simulink model "proc_control"  (R2024b)
settings: Solver=FixedStepAuto  StartTime=0.0  StopTime=inf  RelTol=1e-3
InitFcn:
  | InitProcControl;
model workspace (MAT data in the model file):
  SL_ROS_VariableLengthArrays_MaxSizes : object (value not decoded)
values from neighbouring files (symbols this model uses):
  A = T200Spec16V{:,3}    [InitProcControl.m]
  dmax = simulation.drift.nominal .* rand(1,6)    [InitProcControl.m]
  dmin = -simulation.drift.nominal .* rand(1,6)    [InitProcControl.m]
  dSeedX = round(rand*10)    [InitProcControl.m]
  dts = 5    [InitProcControl.m]
  N = T200Spec16V{:,6}    [InitProcControl.m]
  PWM = T200Spec16V{:,1}    [InitProcControl.m]
  RPM = T200Spec16V{:,2}    [InitProcControl.m]
undefined symbols (not defined in the file or in its folder): angular_velocity, current_gains, data, data_SL_Info, DiscIntNeverNeededParam, elevation, heading, is_mpc_alive, is_trajectory_done, linear_acceleration, motor1, motor2, motor3, motor4, motor5, motor6, motor7, motor8, MPC, mpc_mode, mpc_status, orientation, physics, pose, position, simulation, simulink, target_reached, thrusters_status, thrusters_status_SL_Info, twist, x_vel_btm, y_vel_btm, z_vel_btm
libraries: ros2lib x85, aerolibutil x12, simulink x9, mpclib x3, embmathops x2, sharedtransform x2, robotcorelib x2, sharedTrackingLibrary x1
(part 3 of 3)

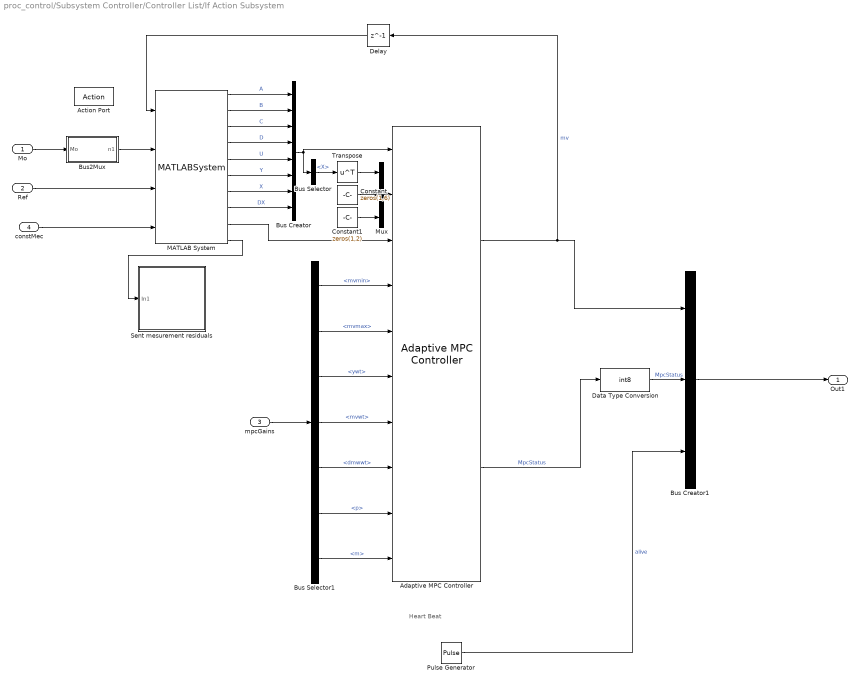
== system proc_control/Subsystem Controller/Controller List/If Action Subsystem ==
  note: Heart Beat
  Mo : Inport
  Ref : Inport  Port=2
  mpcGains : Inport  Port=3
  constMec : Inport  Port=4
  Action Port : ActionPort  InitializeStates=reset  PropagateVarSize=During execution  ActionPortLabel=case [ 10 11 19 31 ]:
  Adaptive MPC Controller : mpclib/Adaptive MPC Controller  SCDEnableBlockLinearizationSpecification=on  mpcobj=Qmpcobj  enable_value=0  updateMPCinCallerWorkspace=on  md_inport=off  mv_inport=off  uref_inport=off  return_cost=off  return_mvseq=off  return_qpstatus=on  return_xseq=off  return_state=off  return_ovseq=off  state_inport=on  isltv_plant=off  umin_inport=on  umax_inport=on  ymin_inport=off  ymax_inport=off  cc_inport=off  ywt_inport=on  uwt_inport=on  duwt_inport=on  rhoeps_inport=off  pm_inport=on  MaximumP=10  HorizonChoice=VariableHorizon  BlockDataType=double  SampleTimeInherited=off  switch_inport=off
  Bus Creator : BusCreator  Inputs=8
  Bus Creator1 : BusCreator  Inputs=3
  Bus Selector : BusSelector  OutputSignals=X
  Bus Selector1 : BusSelector  OutputSignals=mvmin,mvmax,ywt,mvwt,dmwwt,p,m
  Bus2Mux : Subsystem
  Constant : Constant  Value=zeros(1,6)
  Constant1 : Constant  Value=zeros(1,2)
  Data Type Conversion : DataTypeConversion  OutDataTypeStr=int8  SaturateOnIntegerOverflow=off  RndMeth=Floor
  Delay : Delay  DelayLength=1  InitialCondition=zeros(MPC.nu,1)  SampleTime=MPC.Ts
  MATLAB System : MATLABSystem  System=TrimPlant  MPC=MPC  useDynamicsConst=on  SimulateUsing=Code generation
      mask Type: TrimPlant
      mask Display:
      | disp('TrimPlant');
      | port_label('input',1,'u');
      | port_label('input',2,'y');
      | port_label('input',3,'ref');
      | port_label('input',4,'constMec');
      | port_label('output',1,'A');
      | port_label('output',2,'B');
      | port_label('output',3,'C');
      | port_label('output',4,'D');
      | port_label('output',5,'U');
      | port_label('output',6,'Y');
      | port_label('output',7,'X');
      | port_label('output',8,'DX');
      | port_label('output',9,'ref');
      | port_label('output',10,'Z');
  Mux : Mux  Inputs=3
  Pulse Generator : DiscretePulseGenerator  SampleTime=MPC.Ts
  Sent mesurement residuals : Subsystem
  Transpose : Math  Operator=transpose
  Out1 : Outport
  wires:
  Mo/1 -> Bus2Mux/1(Mo)
  Bus2Mux/1(n1) -> MATLAB System/2
  Ref/1 -> MATLAB System/3
  constMec/1 -> MATLAB System/4
  MATLAB System/1 -> Bus Creator/1  "A"
  MATLAB System/2 -> Bus Creator/2  "B"
  MATLAB System/3 -> Bus Creator/3  "C"
  MATLAB System/4 -> Bus Creator/4  "D"
  MATLAB System/5 -> Bus Creator/5  "U"
  MATLAB System/6 -> Bus Creator/6  "Y"
  MATLAB System/7 -> Bus Creator/7  "X"
  MATLAB System/8 -> Bus Creator/8  "DX"
  Bus Creator/1 -> Bus Selector/1, Adaptive MPC Controller/1
  Constant/1 -> Mux/2
  Constant1/1 -> Mux/3
  Mux/1 -> Adaptive MPC Controller/2
  Bus Selector/1 -> Transpose/1  "<X>"
  Transpose/1 -> Mux/1
  MATLAB System/9 -> Adaptive MPC Controller/3
  mpcGains/1 -> Bus Selector1/1
  Bus Selector1/1 -> Adaptive MPC Controller/4  "<mvmin>"
  Bus Selector1/2 -> Adaptive MPC Controller/5  "<mvmax>"
  Bus Selector1/3 -> Adaptive MPC Controller/6  "<ywt>"
  Bus Selector1/4 -> Adaptive MPC Controller/7  "<mvwt>"
  Bus Selector1/5 -> Adaptive MPC Controller/8  "<dmwwt>"
  Bus Selector1/6 -> Adaptive MPC Controller/9  "<p>"
  Bus Selector1/7 -> Adaptive MPC Controller/10  "<m>"
  MATLAB System/10 -> Sent mesurement residuals/1(In1)
  Adaptive MPC Controller/1 -> Delay/1, Bus Creator1/1  "mv"
  Adaptive MPC Controller/2 -> Data Type Conversion/1  "MpcStatus"
  Pulse Generator/1 -> Bus Creator1/3  "alive"
  Delay/1 -> MATLAB System/1
  Bus Creator1/1 -> Out1/1
  Data Type Conversion/1 -> Bus Creator1/2  "MpcStatus"

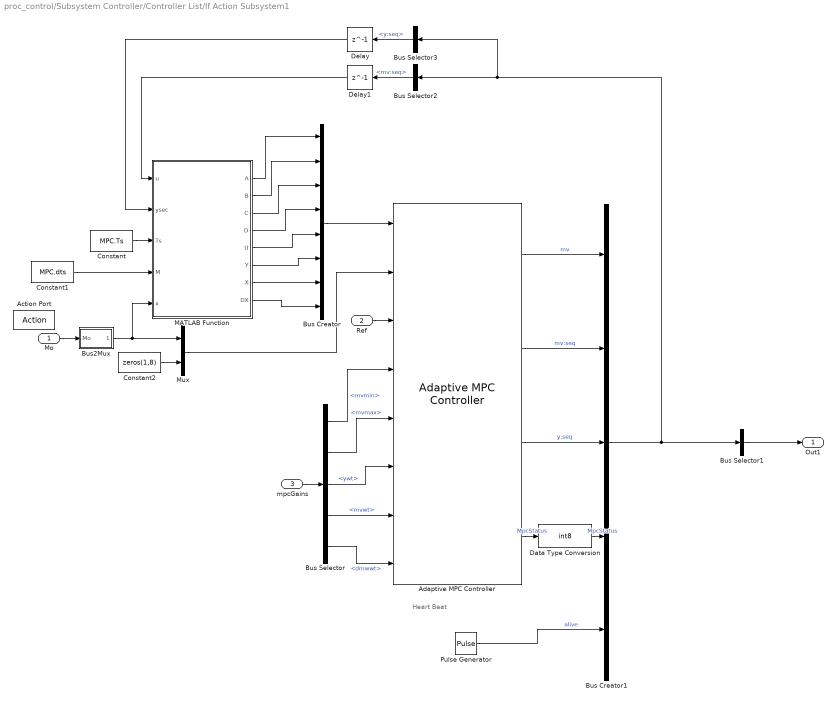
== system proc_control/Subsystem Controller/Controller List/If Action Subsystem1 ==
  note: Heart Beat
  Mo : Inport
  Ref : Inport  Port=2
  mpcGains : Inport  Port=3
  Action Port : ActionPort  InitializeStates=reset  PropagateVarSize=During execution  ActionPortLabel=case [ 30 ]:
  Adaptive MPC Controller : mpclib/Adaptive MPC Controller  SCDEnableBlockLinearizationSpecification=on  mpcobj=Qmpcobj  enable_value=0  updateMPCinCallerWorkspace=on  md_inport=off  mv_inport=off  uref_inport=off  return_cost=off  return_mvseq=on  return_qpstatus=on  return_xseq=off  return_state=off  return_ovseq=on  state_inport=on  isltv_plant=on  umin_inport=on  umax_inport=on  ymin_inport=off  ymax_inport=off  cc_inport=off  ywt_inport=on  uwt_inport=on  duwt_inport=on  rhoeps_inport=off  pm_inport=off  MaximumP=10  HorizonChoice=FixedHorizon  BlockDataType=double  SampleTimeInherited=off  switch_inport=off
  Bus Creator : BusCreator  Inputs=8
  Bus Creator1 : BusCreator  Inputs=5
  Bus Selector : BusSelector  OutputSignals=mvmin,mvmax,ywt,mvwt,dmwwt
  Bus Selector1 : BusSelector  OutputSignals=mv,MpcStatus,alive  OutputAsBus=on
  Bus Selector2 : BusSelector  OutputSignals=mv:seq
  Bus Selector3 : BusSelector  OutputSignals=y:seq
  Bus2Mux : Subsystem
  Constant : Constant  Value=MPC.Ts
  Constant1 : Constant  Value=MPC.dts
  Constant2 : Constant  Value=zeros(1,8)
  Data Type Conversion : DataTypeConversion  OutDataTypeStr=int8  SaturateOnIntegerOverflow=off  RndMeth=Floor
  Delay : Delay  DelayLength=1  InitialCondition=repmat(MPC.Xi.',11,1)  SampleTime=MPC.Ts
  Delay1 : Delay  DelayLength=1  InitialCondition=zeros(11,8)  SampleTime=MPC.Ts
  MATLAB Function : MATLAB Function  TreatAsAtomicUnit=on
  Mux : Mux  Inputs=2
  Pulse Generator : DiscretePulseGenerator  SampleTime=MPC.Ts
  Out1 : Outport
  wires:
  MATLAB Function/2(B) -> Bus Creator/2
  Mo/1 -> Bus2Mux/1(Mo)
  Constant/1 -> MATLAB Function/3(Ts)
  Constant1/1 -> MATLAB Function/4(M)
  Bus Selector/5 -> Adaptive MPC Controller/8  "<dmwwt>"
  MATLAB Function/7(X) -> Bus Creator/7
  Bus2Mux/1(Out1) -> Mux/1, MATLAB Function/5(x)
  Constant2/1 -> Mux/2
  MATLAB Function/3(C) -> Bus Creator/3
  MATLAB Function/1(A) -> Bus Creator/1
  Ref/1 -> Adaptive MPC Controller/3
  Mux/1 -> Adaptive MPC Controller/2
  MATLAB Function/4(D) -> Bus Creator/4
  MATLAB Function/5(U) -> Bus Creator/5
  MATLAB Function/6(Y) -> Bus Creator/6
  MATLAB Function/8(DX) -> Bus Creator/8
  mpcGains/1 -> Bus Selector/1
  Bus Creator/1 -> Adaptive MPC Controller/1
  Bus Selector/2 -> Adaptive MPC Controller/5  "<mvmax>"
  Bus Selector/1 -> Adaptive MPC Controller/4  "<mvmin>"
  Bus Selector/3 -> Adaptive MPC Controller/6  "<ywt>"
  Bus Selector/4 -> Adaptive MPC Controller/7  "<mvwt>"
  Adaptive MPC Controller/1 -> Bus Creator1/1  "mv"
  Adaptive MPC Controller/4 -> Data Type Conversion/1  "MpcStatus"
  Adaptive MPC Controller/3 -> Bus Creator1/3  "y:seq"
  Adaptive MPC Controller/2 -> Bus Creator1/2  "mv:seq"
  Pulse Generator/1 -> Bus Creator1/5  "alive"
  Bus Selector1/1 -> Out1/1
  Bus Creator1/1 -> Bus Selector3/1, Bus Selector2/1, Bus Selector1/1
  Bus Selector3/1 -> Delay/1  "<y:seq>"
  Bus Selector2/1 -> Delay1/1  "<mv:seq>"
  Delay1/1 -> MATLAB Function/1(u)
  Delay/1 -> MATLAB Function/2(ysec)
  Data Type Conversion/1 -> Bus Creator1/4  "MpcStatus"

== system proc_control/Subsystem Controller/Controller List/If Action Subsystem2 ==
  mo : Inport
  ref : Inport  Port=2
  mode : Inport  Port=3
  Action Port : ActionPort  ActionPortLabel=case [ 20 21 ]:
  Bus Creator : BusCreator  Inputs=3
  Constant : Constant  Value=int8(0)
  Constant1 : Constant  Value=0
  Discrete Derivative : simulink/Discrete/Discrete Derivative  gainval=1.0  ICPrevScaledInput=0.0  OutMin=[]  OutMax=[]  OutDataType=fixdt(1, 16)  OutScaling=2^-10  DoSatur=off
  MATLAB System : MATLABSystem  System=OpenLoopController  k=40  binv=binv  mass=physics.mass  volume=physics.volume  height=physics.height  I=physics.I  RG=physics.RG  RB=physics.RB  AddedMass=physics.AddedMass  CDL=physics.CDL  CDQ=physics.CDQ  AF=physics.AF  g=physics.g  rho=physics.rho  SimulateUsing=Code generation
      mask Type: OpenLoopController
      mask Display:
      | disp('OpenLoopController');
      | port_label('input',1,'ref');
      | port_label('input',2,'ref_dot');
      | port_label('input',3,'mo');
      | port_label('input',4,'mode');
      | port_label('output',1,'mv');
  Reshape : Reshape
  Selector : Selector  NumberOfDimensions=2  InputPortWidth=3  IndexOptions=Index vector (dialog),Index vector (dialog)  Indices=1,[8:13]  OutputSizes=1,1
  Out1 : Outport
  wires:
  mode/1 -> MATLAB System/4
  ref/1 -> Selector/1
  Selector/1 -> MATLAB System/1, Discrete Derivative/1
  Discrete Derivative/1 -> MATLAB System/2
  Reshape/1 -> Bus Creator/1  "mv"
  MATLAB System/1 -> Reshape/1
  mo/1 -> MATLAB System/3
  Constant/1 -> Bus Creator/2  "MpcStatus"
  Constant1/1 -> Bus Creator/3  "alive"
  Bus Creator/1 -> Out1/1

== system proc_control/Subsystem Controller/Controller List/If Action Subsystem3 ==
  Action Port : ActionPort  ActionPortLabel=default:
  Bus Creator : BusCreator  Inputs=3
  Constant : Constant  Value=zeros(1,MPC.nu)
  Constant1 : Constant  Value=int8(0)
  Constant2 : Constant  Value=0
  Out1 : Outport
  wires:
  Constant/1 -> Bus Creator/1  "mv"
  Constant1/1 -> Bus Creator/2  "MpcStatus"
  Constant2/1 -> Bus Creator/3  "alive"
  Bus Creator/1 -> Out1/1

== system proc_control/Subsystem Controller/Controller List/Quaternion Non linear MPC (Not for codegen) ==
  note: Heart beat
  Mo : Inport
  Ref : Inport  Port=2
  mpc Gains : Inport  Port=3
  Action Port : ActionPort  InitializeStates=reset  ActionPortLabel=case [ 40 ]:
  Bus Creator : BusCreator  Inputs=3
  Bus Selector : BusSelector  OutputSignals=mvmin,mvmax,ywt,mvwt,dmwwt
  Bus2Mux1 : Subsystem
  Data Type Conversion : DataTypeConversion  OutDataTypeStr=int8  SaturateOnIntegerOverflow=off  RndMeth=Floor
  Delay : Delay  DelayLength=1  InitialCondition=zeros(MPC.nu,1)
  Nonlinear MPC Controller : mpclib/Nonlinear MPC Controller  nlmpcobj=nlobj  UseObjectTs=on  TsControl=0.02  UseMEX=off  md_enabled=off  mvtarget_enabled=off  param_enabled=off  cost_enabled=off  mvseq_enabled=off  stateseq_enabled=off  ovseq_enabled=off  slack_enabled=off  status_enabled=on  ov_min=off  ov_max=off  mv_min=on  mv_max=on  mvrate_min=off  mvrate_max=off  state_min=off  state_max=off  ov_weight=on  mv_weight=on  mvrate_weight=on  ecr_weight=off  nlp_initialize=off
  Pulse Generator : DiscretePulseGenerator  Period=20  PulseWidth=10  SampleTime=MPC.Ts
  Out : Outport
  wires:
  Mo/1 -> Bus2Mux1/1(Mo)
  Bus2Mux1/1(Out1) -> Nonlinear MPC Controller/1
  Ref/1 -> Nonlinear MPC Controller/2
  mpc Gains/1 -> Bus Selector/1
  Bus Selector/1 -> Nonlinear MPC Controller/4  "<mvmin>"
  Bus Selector/2 -> Nonlinear MPC Controller/5  "<mvmax>"
  Bus Selector/3 -> Nonlinear MPC Controller/6  "<ywt>"
  Bus Selector/4 -> Nonlinear MPC Controller/7  "<mvwt>"
  Bus Selector/5 -> Nonlinear MPC Controller/8  "<dmwwt>"
  Nonlinear MPC Controller/1 -> Bus Creator/1, Delay/1  "mv"
  Delay/1 -> Nonlinear MPC Controller/3
  Nonlinear MPC Controller/2 -> Data Type Conversion/1  "MpcStatus"
  Pulse Generator/1 -> Bus Creator/3  "alive"
  Bus Creator/1 -> Out/1
  Data Type Conversion/1 -> Bus Creator/2  "MpcStatus"

== system proc_control/Subsystem Controller/If Action Subsystem/Subsystem ==
  Bus Creator : BusCreator  Inputs=8
  Constant : Constant  Value=zeros(1, 128)
  Constant1 : Constant  Value=zeros(1, 128)
  Constant2 : Constant  Value=zeros(1, 128)
  Constant3 : Constant  Value=MPC.tmax
  Constant4 : Constant  Value=MPC.tmin
  Subsystem : Subsystem
  Subsystem1 : Subsystem
  Subsystem2 : Subsystem
  Out1 : Outport
  wires:
  Constant4/1 -> Bus Creator/8  "min_thrust"
  Constant2/1 -> Bus Creator/5  "mvr"
  Constant3/1 -> Bus Creator/7  "max_thrust"
  Constant/1 -> Bus Creator/1  "ov"
  Subsystem/1(Out1) -> Bus Creator/2  "ov_SL_Info"
  Subsystem2/1(Out1) -> Bus Creator/4  "mv_SL_Info"
  Constant1/1 -> Bus Creator/3  "mv"
  Subsystem1/1(Out1) -> Bus Creator/6  "mvr_SL_Info"
  Bus Creator/1 -> Out1/1

== system proc_control/Subsystem ProcNav/DVL Measurements/DVL2Ship ==
  dvl Rotation : Inport
  Constant : Constant  Value=0
  Delay : Delay  DelayLength=1  InitialCondition=1
  Enabled Subsystem : Subsystem  TreatAsAtomicUnit=on
  Quat : Outport
  wires:
  Constant/1 -> Delay/1
  Delay/1 -> Enabled Subsystem/Enable
  dvl Rotation/1 -> Enabled Subsystem/1(dvl Rotation)
  Enabled Subsystem/1(Quat) -> Quat/1

== system proc_control/Subsystem ProcNav/SLAM Measurements/Subsystem ==
  VisData : Inport
  Blank Message : ros2lib/Blank Message  messageClass=Message  entityType=nav_msgs/Odometry  messageType=nav_msgs/Odometry  SampleTime=inf
  Bus Assignment : BusAssignment  AssignedSignals=pose.pose.position.x,pose.pose.position.y,pose.pose.position.z,pose.pose.orientation.w,pose.pose.orientation.x,pose.pose.orientation.y,pose.pose.orientation.z,twist.twist.linear.x,twist.twist.linear.y,twist.twist.linear.z,twist.twist.angular.x,twist.twist.angular.y,twist.twist.angular.z
  Demux : Demux  Outputs=13
  Header Assignment : ros2lib/Header Assignment  SetFrameID=off  InsertTimeStamp=on  SetHeaderFieldName=Use the default header field name  HeaderFieldName=header
  Publish : ros2lib/Publish  topicSource=Specify your own  topic=/proc_nav/slam/vis  messageType=nav_msgs/Odometry  QOSHistory=Keep last  QOSDepth=1  QOSReliability=Reliable  QOSDurability=Volatile  QOSDeadline=Inf  QOSLifespan=Inf  QOSLiveliness=Automatic  QOSLeaseDuration=Inf  QOSAvoidROSNamespaceConventions=off
  wires:
  Demux/8 -> Bus Assignment/9
  Demux/10 -> Bus Assignment/11
  Blank Message/1 -> Header Assignment/1
  Demux/6 -> Bus Assignment/7
  Demux/2 -> Bus Assignment/3
  Bus Assignment/1 -> Publish/1
  Demux/9 -> Bus Assignment/10
  Demux/13 -> Bus Assignment/14
  Demux/5 -> Bus Assignment/6
  Demux/7 -> Bus Assignment/8
  VisData/1 -> Demux/1
  Demux/3 -> Bus Assignment/4
  Header Assignment/1 -> Bus Assignment/1
  Demux/4 -> Bus Assignment/5
  Demux/12 -> Bus Assignment/13
  Demux/1 -> Bus Assignment/2
  Demux/11 -> Bus Assignment/12

== system proc_control/Subsystem ProcNav/SLAM Measurements/Subsystem1 ==
  TrackingData : Inport
  Blank Message : ros2lib/Blank Message  messageClass=Message  entityType=nav_msgs/Odometry  messageType=nav_msgs/Odometry  SampleTime=inf
  Bus Assignment : BusAssignment  AssignedSignals=pose.pose.position.x,pose.pose.position.y,pose.pose.position.z,pose.pose.orientation.w,pose.pose.orientation.x,pose.pose.orientation.y,pose.pose.orientation.z,twist.twist.linear.x,twist.twist.linear.y,twist.twist.linear.z,twist.twist.angular.x,twist.twist.angular.y,twist.twist.angular.z
  Demux : Demux  Outputs=13
  Header Assignment : ros2lib/Header Assignment  SetFrameID=off  InsertTimeStamp=on  SetHeaderFieldName=Use the default header field name  HeaderFieldName=header
  Publish : ros2lib/Publish  topicSource=Specify your own  topic=/proc_nav/slam/tracking  messageType=nav_msgs/Odometry  QOSHistory=Keep last  QOSDepth=1  QOSReliability=Reliable  QOSDurability=Volatile  QOSDeadline=Inf  QOSLifespan=Inf  QOSLiveliness=Automatic  QOSLeaseDuration=Inf  QOSAvoidROSNamespaceConventions=off
  wires:
  Demux/8 -> Bus Assignment/9
  Demux/10 -> Bus Assignment/11
  Blank Message/1 -> Header Assignment/1
  Demux/6 -> Bus Assignment/7
  Demux/2 -> Bus Assignment/3
  Bus Assignment/1 -> Publish/1
  Demux/9 -> Bus Assignment/10
  Demux/13 -> Bus Assignment/14
  Demux/5 -> Bus Assignment/6
  Demux/7 -> Bus Assignment/8
  TrackingData/1 -> Demux/1
  Demux/3 -> Bus Assignment/4
  Header Assignment/1 -> Bus Assignment/1
  Demux/4 -> Bus Assignment/5
  Demux/12 -> Bus Assignment/13
  Demux/1 -> Bus Assignment/2
  Demux/11 -> Bus Assignment/12

== system proc_control/Subsystem Trajectory/singleWpts Trajectory Control DEBUG only/Enabled Subsystem ==
  In1 : Inport
  Enable : EnablePort
  Bus Selector : BusSelector  OutputSignals=frame,speed  OutputAsBus=on
  Bus Selector1 : BusSelector  OutputSignals=position.x,position.y,position.z,orientation.z,orientation.y,orientation.x  OutputAsBus=on
  Bus Selector2 : BusSelector  OutputSignals=fine  OutputAsBus=on
  Data Type Conversion : DataTypeConversion  OutDataTypeStr=double  SaturateOnIntegerOverflow=off  RndMeth=Floor  LockScale=on
  Data Type Conversion1 : DataTypeConversion  OutDataTypeStr=double  SaturateOnIntegerOverflow=off  RndMeth=Floor  LockScale=on
  Data Type Conversion2 : DataTypeConversion  OutDataTypeStr=double  SaturateOnIntegerOverflow=off  RndMeth=Floor  LockScale=on
  Mux : Mux  Inputs=3
  Out1 : Outport
  wires:
  In1/1 -> Bus Selector2/1, Bus Selector1/1, Bus Selector/1
  Bus Selector1/1 -> Data Type Conversion/1
  Bus Selector2/1 -> Data Type Conversion2/1
  Bus Selector/1 -> Data Type Conversion1/1
  Mux/1 -> Out1/1
  Data Type Conversion/1 -> Mux/1
  Data Type Conversion1/1 -> Mux/2
  Data Type Conversion2/1 -> Mux/3

== system proc_control/Subsystem Trajectory/singleWpts Trajectory Control DEBUG only/Pre-traitement ==
  In1 : Inport
  Enable : EnablePort
  Constant : Constant  Value=0
  Display : Display
  Matrix Concatenate : Concatenate  Mode=Multidimensional array
  Selector : Selector  NumberOfDimensions=2  InputPortWidth=3  IndexOptions=Index vector (dialog),Index vector (dialog)  Indices=[1:3],[1:2]  OutputSizes=1,1
  Selector1 : Selector  NumberOfDimensions=2  InputPortWidth=3  IndexOptions=Index vector (dialog),Index vector (dialog)  Indices=[4:7],[1:2]  OutputSizes=1,1
  Selector2 : Selector  NumberOfDimensions=2  InputPortWidth=3  IndexOptions=Index vector (dialog),Index vector (dialog)  Indices=[8],[2]  OutputSizes=1,1
  Selector3 : Selector  NumberOfDimensions=2  InputPortWidth=3  IndexOptions=Index vector (dialog),Index vector (dialog)  Indices=[9],[2]  OutputSizes=1,1
  Selector4 : Selector  NumberOfDimensions=2  InputPortWidth=3  IndexOptions=Index vector (dialog),Index vector (dialog)  Indices=[1:7],[2]  OutputSizes=1,1
  Terminator : Terminator
  Transpose : Math  Operator=transpose
  linWpts : Outport
  RotWpts : Outport  Port=2
  time : Outport  Port=3
  target : Outport  Port=4
  wires:
  In1/1 -> Transpose/1
  Transpose/1 -> Display/1, Selector4/1, Selector3/1, Selector2/1, Selector1/1, Selector/1
  Selector/1 -> linWpts/1
  Selector1/1 -> RotWpts/1
  Constant/1 -> Matrix Concatenate/1
  Selector2/1 -> Matrix Concatenate/2
  Matrix Concatenate/1 -> time/1
  Selector3/1 -> Terminator/1
  Selector4/1 -> target/1

== system proc_control/Subsystem Trajectory/singleWpts Trajectory Control DEBUG only/Resettable Subsystem ==
  linWpts : Inport
  rotWpts : Inport  Port=2
  time : Inport  Port=3
  Reset : ResetPort  DisableCoverage=on
  Constant : Constant
  Discrete-Time Integrator : DiscreteIntegrator  IntegratorMethod=Integration: Trapezoidal  SampleTime=-1  ICPrevOutput=DiscIntNeverNeededParam  ICPrevScaledInput=DiscIntNeverNeededParam
  Rotation Trajectory : robotcorelib/Rotation Trajectory  WaypointFormat=Quaternion  WaypointSource=External  R0=[ 1, 0, 0, 0 ]'  RF=[ 0, 0, 1, 0 ]'  TimeInterval=[ 0, 1 ]  CustomTimeScaling=off  ParameterSource=Internal  TSTime=0:0.1:1  TimeScaling=[ 0:0.1:1; ones( 1, 11 ); zeros( 1, 11 ) ]  SimulateUsing=Code generation
      settings: LibrarySourceBlock=robotutilslib/Rotation Trajectory
  Selector : Selector  NumberOfDimensions=2  InputPortWidth=3  IndexOptions=Index vector (dialog),Index vector (dialog)  Indices=[1:4],1  OutputSizes=1,1
  Selector1 : Selector  NumberOfDimensions=2  InputPortWidth=3  IndexOptions=Index vector (dialog),Index vector (dialog)  Indices=[1:4],1  OutputSizes=1,1
  Subsystem : Subsystem
  Terminator : Terminator
  n1 : Outport
  epsilon : Outport  Port=2
  v1 : Outport  Port=3
  v2 : Outport  Port=4
  wires:
  Rotation Trajectory/3 -> Terminator/1
  time/1 -> Subsystem/3(time), Rotation Trajectory/4
  Constant/1 -> Discrete-Time Integrator/1
  linWpts/1 -> Subsystem/2(linWpts)
  Rotation Trajectory/1 -> epsilon/1
  Selector1/1 -> Rotation Trajectory/3
  Subsystem/1(n1) -> n1/1
  rotWpts/1 -> Selector1/1, Selector/1
  Discrete-Time Integrator/1 -> Rotation Trajectory/1, Subsystem/1(In1)
  Rotation Trajectory/2 -> v2/1
  Selector/1 -> Rotation Trajectory/2
  Subsystem/2(v1) -> v1/1

== system proc_control/Subsystem Trajectory/singleWpts Trajectory Control DEBUG only/Subsystem ==
  Bus Creator : BusCreator  Inputs=3
  Bus Creator1 : BusCreator  Inputs=3
  Bus Creator2 : BusCreator  Inputs=6
  Constant{1..6} (6 alike) : Constant  Value=0
  Frame : Constant
  fine : Constant
  speed : Constant
  speed1 : Constant
  Out1 : Outport
  wires:
  Constant4/1 -> Bus Creator/1  "x"
  Constant6/1 -> Bus Creator1/1  "x"
  Bus Creator1/1 -> Bus Creator2/4  "orientation"
  Constant2/1 -> Bus Creator/2  "y"
  Constant3/1 -> Bus Creator/3  "z"
  Frame/1 -> Bus Creator2/1  "frame"
  Constant1/1 -> Bus Creator1/2  "y"
  Constant5/1 -> Bus Creator1/3  "z"
  speed/1 -> Bus Creator2/2  "speed"
  Bus Creator/1 -> Bus Creator2/3  "position"
  fine/1 -> Bus Creator2/5  "fine"
  speed1/1 -> Bus Creator2/6  "rotation"
  Bus Creator2/1 -> Out1/1

== system proc_control/Model System/Sensor Model/Hydrophones Model/If Action Subsystem ==
  In1 : Inport
  Action Port : ActionPort  ActionPortLabel=if(u1 == 0)
  Out1 : Outport
  wires:
  In1/1 -> Out1/1

== system proc_control/Ros Command/Get_ROS_param/MPC Parameters/MPC Gains ==
  Bus Creator : BusCreator  Inputs=9
  Data Type Conversion : DataTypeConversion  OutDataTypeStr=double  SaturateOnIntegerOverflow=off  RndMeth=Floor
  Data Type Conversion1 : DataTypeConversion  OutDataTypeStr=double  SaturateOnIntegerOverflow=off  RndMeth=Floor
  Gains Default : Subsystem
  Gains Mode 10 : Subsystem
  Gains Mode 11 : Subsystem
  Gains Mode 19 : Subsystem
  Gains No DVL : Subsystem
  M : ros2lib/Get Parameter  ParameterName=proc_control.mpc.m  ParameterType=int64  ParameterMaxArrayLength=64  ParameterInitialValue=MPC.m  SampleTime=-1  ModelName=proc_control  BlockId=ParamGet_proc_control_143
  P : ros2lib/Get Parameter  ParameterName=proc_control.mpc.p  ParameterType=int64  ParameterMaxArrayLength=64  ParameterInitialValue=MPC.p  SampleTime=-1  ModelName=proc_control  BlockId=ParamGet_proc_control_140
  T Max : ros2lib/Get Parameter  ParameterName=proc_control.mpc.tmax  ParameterType=double  ParameterMaxArrayLength=64  ParameterInitialValue=MPC.tmax  SampleTime=-1  ModelName=proc_control  BlockId=ParamGet_proc_control_144
  T Min : ros2lib/Get Parameter  ParameterName=proc_control.mpc.tmin  ParameterType=double  ParameterMaxArrayLength=64  ParameterInitialValue=MPC.tmin  SampleTime=-1  ModelName=proc_control  BlockId=ParamGet_proc_control_145
  gains : Outport
  wires:
  P/1 -> Data Type Conversion/1  "p"
  Gains Mode 11/1(c11) -> Bus Creator/3
  M/1 -> Data Type Conversion1/1  "m"
  Data Type Conversion/1 -> Bus Creator/6  "p"
  Gains Default/1(default) -> Bus Creator/1
  Gains Mode 10/1(c10) -> Bus Creator/2
  Gains No DVL/1(noDvl) -> Bus Creator/5
  Gains Mode 19/1(c19) -> Bus Creator/4
  Data Type Conversion1/1 -> Bus Creator/7  "m"
  T Max/1 -> Bus Creator/8  "tmax"
  T Min/1 -> Bus Creator/9  "tmin"
  Bus Creator/1 -> gains/1  "gains"

== system proc_control/Ros Command/Get_ROS_param/MPC Parameters/targetReached Params ==
  Angular Tolerance : ros2lib/Get Parameter  ParameterName=proc_control.target_reached.angular_tolerance  ParameterType=double  ParameterMaxArrayLength=16  ParameterInitialValue=MPC.targetReached.angularTol  SampleTime=-1  ModelName=proc_control  BlockId=ParamGet_proc_control_151
  Bus Creator : BusCreator  Inputs=3
  Linear Tolerance : ros2lib/Get Parameter  ParameterName=proc_control.target_reached.linear_tolerance  ParameterType=double  ParameterMaxArrayLength=16  ParameterInitialValue=MPC.targetReached.linearTol  SampleTime=-1  ModelName=proc_control  BlockId=ParamGet_proc_control_150
  Time In Tolerance : ros2lib/Get Parameter  ParameterName=proc_control.target_reached.time_in_tolerance  ParameterType=double  ParameterMaxArrayLength=16  ParameterInitialValue=MPC.targetReached.timeInTol  SampleTime=-1  ModelName=proc_control  BlockId=ParamGet_proc_control_152
  targetReached : Outport
  wires:
  Linear Tolerance/1 -> Bus Creator/1  "linearTol"
  Angular Tolerance/1 -> Bus Creator/2  "angularTol"
  Time In Tolerance/1 -> Bus Creator/3  "timeInTol"
  Bus Creator/1 -> targetReached/1  "targetReached"

== system proc_control/Subsystem Controller/Controller List/If Action Subsystem/Bus2Mux ==
  Mo : Inport
  Bus Selector : BusSelector  OutputSignals=WorldPosition,qS2W,Body Velocity,Angular Rate
  Mux : Mux
  n1 : Outport
  wires:
  Mo/1 -> Bus Selector/1
  Mux/1 -> n1/1
  Bus Selector/2 -> Mux/2  "<qS2W>"
  Bus Selector/1 -> Mux/1  "<WorldPosition>"
  Bus Selector/3 -> Mux/3  "<Body Velocity>"
  Bus Selector/4 -> Mux/4  "<Angular Rate>"

== system proc_control/Subsystem Controller/Controller List/If Action Subsystem/Sent mesurement residuals ==
  In1 : Inport
  Blank Message : ros2lib/Blank Message  messageClass=Message  entityType=nav_msgs/Odometry  messageType=nav_msgs/Odometry  SampleTime=-1
  Bus Assignment : BusAssignment  AssignedSignals=pose.pose.position.x,pose.pose.position.y,pose.pose.position.z,pose.pose.orientation.w,pose.pose.orientation.x,pose.pose.orientation.y,pose.pose.orientation.z,twist.twist.linear.x,twist.twist.linear.y,twist.twist.linear.z,twist.twist.angular.x,twist.twist.angular.y,twist.twist.angular.z
  Demux : Demux  Outputs=13
  Header Assignment : ros2lib/Header Assignment  SetFrameID=on  FrameID=NED  InsertTimeStamp=on  SetHeaderFieldName=Use the default header field name  HeaderFieldName=header
  Publish : ros2lib/Publish  topicSource=Specify your own  topic=/proc_control/measurment_residual  messageType=nav_msgs/Odometry  QOSHistory=Keep last  QOSDepth=1  QOSReliability=Reliable  QOSDurability=Volatile  QOSDeadline=Inf  QOSLifespan=Inf  QOSLiveliness=Automatic  QOSLeaseDuration=Inf  QOSAvoidROSNamespaceConventions=off
  wires:
  Blank Message/1 -> Header Assignment/1
  Header Assignment/1 -> Bus Assignment/1
  Demux/1 -> Bus Assignment/2
  Demux/2 -> Bus Assignment/3
  Demux/3 -> Bus Assignment/4
  Demux/4 -> Bus Assignment/6
  Demux/5 -> Bus Assignment/5
  Demux/6 -> Bus Assignment/7
  Demux/7 -> Bus Assignment/8
  Demux/8 -> Bus Assignment/9
  Demux/9 -> Bus Assignment/10
  Demux/10 -> Bus Assignment/11
  Demux/11 -> Bus Assignment/12
  Demux/12 -> Bus Assignment/13
  Demux/13 -> Bus Assignment/14
  In1/1 -> Demux/1
  Bus Assignment/1 -> Publish/1

== system proc_control/Subsystem Controller/Controller List/If Action Subsystem1/Bus2Mux ==
  Mo : Inport
  Bus Selector : BusSelector  OutputSignals=WorldPosition,qS2W,Body Velocity,Angular Rate
  Mux : Mux
  Out1 : Outport
  wires:
  Mo/1 -> Bus Selector/1
  Bus Selector/1 -> Mux/1  "<WorldPosition>"
  Bus Selector/2 -> Mux/2  "<qS2W>"
  Bus Selector/3 -> Mux/3  "<Body Velocity>"
  Bus Selector/4 -> Mux/4  "<Angular Rate>"
  Mux/1 -> Out1/1

== system proc_control/Subsystem Controller/Controller List/Quaternion Non linear MPC (Not for codegen)/Bus2Mux1 ==
  Mo : Inport
  Bus Selector : BusSelector  OutputSignals=WorldPosition,qS2W,Body Velocity,Angular Rate
  Mux : Mux
  Out1 : Outport
  wires:
  Mo/1 -> Bus Selector/1
  Bus Selector/1 -> Mux/1  "<WorldPosition>"
  Bus Selector/2 -> Mux/2  "<qS2W>"
  Bus Selector/3 -> Mux/3  "<Body Velocity>"
  Bus Selector/4 -> Mux/4  "<Angular Rate>"
  Mux/1 -> Out1/1

== system proc_control/Subsystem Controller/If Action Subsystem/Subsystem/Subsystem ==
  Bus Creator : BusCreator  Inputs=2
  Constant : Constant  Value=uint32(0)
  Constant1 : Constant  Value=uint32(0)
  Out1 : Outport
  wires:
  Constant/1 -> Bus Creator/1  "CurrentLength"
  Bus Creator/1 -> Out1/1
  Constant1/1 -> Bus Creator/2  "ReceivedLength"

== system proc_control/Subsystem Controller/If Action Subsystem/Subsystem/Subsystem1 ==
  Bus Creator : BusCreator  Inputs=2
  Constant : Constant  Value=uint32(0)
  Constant1 : Constant  Value=uint32(0)
  Out1 : Outport
  wires:
  Bus Creator/1 -> Out1/1
  Constant/1 -> Bus Creator/1  "CurrentLength"
  Constant1/1 -> Bus Creator/2  "ReceivedLength"

== system proc_control/Subsystem Controller/If Action Subsystem/Subsystem/Subsystem2 ==
  Bus Creator : BusCreator  Inputs=2
  Constant : Constant  Value=uint32(0)
  Constant1 : Constant  Value=uint32(0)
  Out1 : Outport
  wires:
  Bus Creator/1 -> Out1/1
  Constant/1 -> Bus Creator/1  "CurrentLength"
  Constant1/1 -> Bus Creator/2  "ReceivedLength"

== system proc_control/Subsystem ProcNav/DVL Measurements/DVL2Ship/Enabled Subsystem ==
  dvl Rotation : Inport
  Enable : EnablePort
  Rotation Angles to Quaternions : sharedtransform/Rotation Angles to Quaternions  rotationOrder=XYZ  aMode=aMode
  Quat : Outport
  wires:
  dvl Rotation/1 -> Rotation Angles to Quaternions/1
  Rotation Angles to Quaternions/1 -> Quat/1

== system proc_control/Subsystem Trajectory/singleWpts Trajectory Control DEBUG only/Resettable Subsystem/Subsystem ==
  In1 : Inport
  linWpts : Inport  Port=2
  time : Inport  Port=3
  Polynomial Trajectory : robotcorelib/Polynomial Trajectory  WaypointSource=External  Waypoints=[ 0, 2, 1, 5, 0; -1, 3, 1, 4, 4 ]  TimePoints=[ 0, 1, 2, 3, 4 ]  TimeInterval=[ 1, 4 ]  Method=Cubic Polynomial  ParameterSource=Internal  VelocityBoundaryCondition=zeros( 3, 2 )  AccelerationBoundaryCondition=zeros( 2, 5 )  SimulateUsing=Code generation
  Terminator : Terminator
  n1 : Outport
  v1 : Outport  Port=2
  wires:
  In1/1 -> Polynomial Trajectory/1
  linWpts/1 -> Polynomial Trajectory/2
  time/1 -> Polynomial Trajectory/3
  Polynomial Trajectory/1 -> n1/1
  Polynomial Trajectory/2 -> v1/1
  Polynomial Trajectory/3 -> Terminator/1

== system proc_control/Ros Command/Get_ROS_param/MPC Parameters/MPC Gains/Gains Default ==
  Bus Creator : BusCreator  Inputs=3
  MATLAB System1 : MATLABSystem  System=Vector2DoubleArray  arraySize=[1 MPC.nu]  constantName='Default MVR'  SimulateUsing=Code generation
      mask Type: Vector2DoubleArray
      mask Display:
      | disp('Vector2DoubleArray');
      | port_label('input',1,'vector');
      | port_label('input',2,'length');
      | port_label('output',1,'array');
  MATLAB System3 : MATLABSystem  System=Vector2DoubleArray  arraySize=[1 MPC.nx]  constantName='Default OV'  SimulateUsing=Code generation
      mask Type: Vector2DoubleArray
      mask Display:
      | disp('Vector2DoubleArray');
      | port_label('input',1,'vector');
      | port_label('input',2,'length');
      | port_label('output',1,'array');
  MATLAB System4 : MATLABSystem  System=Vector2DoubleArray  arraySize=[1, MPC.nu]  constantName='Default MV'  SimulateUsing=Code generation
      mask Type: Vector2DoubleArray
      mask Display:
      | disp('Vector2DoubleArray');
      | port_label('input',1,'vector');
      | port_label('input',2,'length');
      | port_label('output',1,'array');
  MV : ros2lib/Get Parameter  ParameterName=proc_control.mpc.gains.default.mv  ParameterType=double[]  ParameterMaxArrayLength=64  ParameterInitialValue=double([30,30,30,45,45,45,45,0])  SampleTime=-1  ModelName=proc_control  BlockId=ParamGet_proc_control_72
  MVR : ros2lib/Get Parameter  ParameterName=proc_control.mpc.gains.default.mvr  ParameterType=double[]  ParameterMaxArrayLength=64  ParameterInitialValue=double([30,30,30,45,45,45,45,0])  SampleTime=-1  ModelName=proc_control  BlockId=ParamGet_proc_control_74
  OV : ros2lib/Get Parameter  ParameterName=proc_control.mpc.gains.default.ov  ParameterType=double[]  ParameterMaxArrayLength=64  ParameterInitialValue=double([30.0,30.0,30.0,45.0,45.0,45.0,45.0,0.0,0.0,0.0,0.0,0.0,0.0])  SampleTime=-1  ModelName=proc_control  BlockId=ParamGet_proc_control_66
  default : Outport
  wires:
  OV/1 -> MATLAB System3/1
  OV/2 -> MATLAB System3/2
  MVR/2 -> MATLAB System1/2
  MV/1 -> MATLAB System4/1
  MATLAB System3/1 -> Bus Creator/1  "OV"
  MV/2 -> MATLAB System4/2
  MATLAB System4/1 -> Bus Creator/2  "MV"
  MVR/1 -> MATLAB System1/1
  MATLAB System1/1 -> Bus Creator/3  "MVR"
  Bus Creator/1 -> default/1  "predefined"

== system proc_control/Ros Command/Get_ROS_param/MPC Parameters/MPC Gains/Gains Mode 10 ==
  Bus Creator : BusCreator  Inputs=3
  MATLAB System3 : MATLABSystem  System=Vector2DoubleArray  arraySize=[1 MPC.nu]  constantName='M10 MVR'  SimulateUsing=Code generation
      mask Type: Vector2DoubleArray
      mask Display:
      | disp('Vector2DoubleArray');
      | port_label('input',1,'vector');
      | port_label('input',2,'length');
      | port_label('output',1,'array');
  MATLAB System4 : MATLABSystem  System=Vector2DoubleArray  arraySize=[1 MPC.nx]  constantName='M10 OV'  SimulateUsing=Code generation
      mask Type: Vector2DoubleArray
      mask Display:
      | disp('Vector2DoubleArray');
      | port_label('input',1,'vector');
      | port_label('input',2,'length');
      | port_label('output',1,'array');
  MATLAB System5 : MATLABSystem  System=Vector2DoubleArray  arraySize=[1 MPC.nu]  constantName='M10 MV'  SimulateUsing=Code generation
      mask Type: Vector2DoubleArray
      mask Display:
      | disp('Vector2DoubleArray');
      | port_label('input',1,'vector');
      | port_label('input',2,'length');
      | port_label('output',1,'array');
  MV : ros2lib/Get Parameter  ParameterName=proc_control.mpc.gains.c10.mv  ParameterType=double[]  ParameterMaxArrayLength=64  ParameterInitialValue=uint8([30,30,30,45,45,45,45,0])  SampleTime=-1  ModelName=proc_control  BlockId=ParamGet_proc_control_98
  MVR : ros2lib/Get Parameter  ParameterName=proc_control.mpc.gains.c10.mvr  ParameterType=double[]  ParameterMaxArrayLength=64  ParameterInitialValue=uint8([30,30,30,45,45,45,45,0])  SampleTime=-1  ModelName=proc_control  BlockId=ParamGet_proc_control_99
  OV : ros2lib/Get Parameter  ParameterName=proc_control.mpc.gains.c10.ov  ParameterType=double[]  ParameterMaxArrayLength=64  ParameterInitialValue=uint8([30,30,30,45,45,45,45,0,0,0,0,0,0])  SampleTime=-1  ModelName=proc_control  BlockId=ParamGet_proc_control_97
  c10 : Outport
  wires:
  OV/1 -> MATLAB System4/1
  OV/2 -> MATLAB System4/2
  MVR/2 -> MATLAB System3/2
  MV/1 -> MATLAB System5/1
  MATLAB System4/1 -> Bus Creator/1  "OV"
  MV/2 -> MATLAB System5/2
  MATLAB System5/1 -> Bus Creator/2  "MV"
  MVR/1 -> MATLAB System3/1
  MATLAB System3/1 -> Bus Creator/3  "MVR"
  Bus Creator/1 -> c10/1  "c10"

== system proc_control/Ros Command/Get_ROS_param/MPC Parameters/MPC Gains/Gains Mode 11 ==
  Bus Creator : BusCreator  Inputs=3
  MATLAB System3 : MATLABSystem  System=Vector2DoubleArray  arraySize=[1 MPC.nu]  constantName='M11 MVR'  SimulateUsing=Code generation
      mask Type: Vector2DoubleArray
      mask Display:
      | disp('Vector2DoubleArray');
      | port_label('input',1,'vector');
      | port_label('input',2,'length');
      | port_label('output',1,'array');
  MATLAB System4 : MATLABSystem  System=Vector2DoubleArray  arraySize=[1 MPC.nx]  constantName='M11 OV'  SimulateUsing=Code generation
      mask Type: Vector2DoubleArray
      mask Display:
      | disp('Vector2DoubleArray');
      | port_label('input',1,'vector');
      | port_label('input',2,'length');
      | port_label('output',1,'array');
  MATLAB System5 : MATLABSystem  System=Vector2DoubleArray  arraySize=[1 MPC.nu]  constantName='M11 MV'  SimulateUsing=Code generation
      mask Type: Vector2DoubleArray
      mask Display:
      | disp('Vector2DoubleArray');
      | port_label('input',1,'vector');
      | port_label('input',2,'length');
      | port_label('output',1,'array');
  MV : ros2lib/Get Parameter  ParameterName=proc_control.mpc.gains.c11.mv  ParameterType=double[]  ParameterMaxArrayLength=64  ParameterInitialValue=uint8([30,30,30,45,45,45,45,0])  SampleTime=-1  ModelName=proc_control  BlockId=ParamGet_proc_control_107
  MVR : ros2lib/Get Parameter  ParameterName=proc_control.mpc.gains.c11.mvr  ParameterType=double[]  ParameterMaxArrayLength=64  ParameterInitialValue=uint8([30,30,30,45,45,45,45,0])  SampleTime=-1  ModelName=proc_control  BlockId=ParamGet_proc_control_108
  OV : ros2lib/Get Parameter  ParameterName=proc_control.mpc.gains.c11.ov  ParameterType=double[]  ParameterMaxArrayLength=64  ParameterInitialValue=uint8([30,30,30,45,45,45,45,0,0,0,0,0,0])  SampleTime=-1  ModelName=proc_control  BlockId=ParamGet_proc_control_106
  c11 : Outport
  wires:
  OV/1 -> MATLAB System4/1
  OV/2 -> MATLAB System4/2
  MVR/2 -> MATLAB System3/2
  MV/1 -> MATLAB System5/1
  MATLAB System4/1 -> Bus Creator/1  "OV"
  MV/2 -> MATLAB System5/2
  MATLAB System5/1 -> Bus Creator/2  "MV"
  MVR/1 -> MATLAB System3/1
  MATLAB System3/1 -> Bus Creator/3  "MVR"
  Bus Creator/1 -> c11/1  "c11"

== system proc_control/Ros Command/Get_ROS_param/MPC Parameters/MPC Gains/Gains Mode 19 ==
  Bus Creator : BusCreator  Inputs=3
  MATLAB System3 : MATLABSystem  System=Vector2DoubleArray  arraySize=[1 MPC.nu]  constantName='M19 MVR'  SimulateUsing=Code generation
      mask Type: Vector2DoubleArray
      mask Display:
      | disp('Vector2DoubleArray');
      | port_label('input',1,'vector');
      | port_label('input',2,'length');
      | port_label('output',1,'array');
  MATLAB System4 : MATLABSystem  System=Vector2DoubleArray  arraySize=[1 MPC.nx]  constantName='M19 OV'  SimulateUsing=Code generation
      mask Type: Vector2DoubleArray
      mask Display:
      | disp('Vector2DoubleArray');
      | port_label('input',1,'vector');
      | port_label('input',2,'length');
      | port_label('output',1,'array');
  MATLAB System5 : MATLABSystem  System=Vector2DoubleArray  arraySize=[1 MPC.nu]  constantName='M19 MV'  SimulateUsing=Code generation
      mask Type: Vector2DoubleArray
      mask Display:
      | disp('Vector2DoubleArray');
      | port_label('input',1,'vector');
      | port_label('input',2,'length');
      | port_label('output',1,'array');
  MV : ros2lib/Get Parameter  ParameterName=proc_control.mpc.gains.c19.mv  ParameterType=double[]  ParameterMaxArrayLength=64  ParameterInitialValue=uint8([30,30,30,45,45,45,45,0])  SampleTime=-1  ModelName=proc_control  BlockId=ParamGet_proc_control_116
  MVR : ros2lib/Get Parameter  ParameterName=proc_control.mpc.gains.c19.mvr  ParameterType=double[]  ParameterMaxArrayLength=64  ParameterInitialValue=uint8([30,30,30,45,45,45,45,0])  SampleTime=-1  ModelName=proc_control  BlockId=ParamGet_proc_control_117
  OV : ros2lib/Get Parameter  ParameterName=proc_control.mpc.gains.c19.ov  ParameterType=double[]  ParameterMaxArrayLength=64  ParameterInitialValue=uint8([30,30,30,45,45,45,45,0,0,0,0,0,0])  SampleTime=-1  ModelName=proc_control  BlockId=ParamGet_proc_control_115
  c19 : Outport
  wires:
  OV/1 -> MATLAB System4/1
  OV/2 -> MATLAB System4/2
  MVR/2 -> MATLAB System3/2
  MV/1 -> MATLAB System5/1
  MATLAB System4/1 -> Bus Creator/1  "OV"
  MV/2 -> MATLAB System5/2
  MATLAB System5/1 -> Bus Creator/2  "MV"
  MVR/1 -> MATLAB System3/1
  MATLAB System3/1 -> Bus Creator/3  "MVR"
  Bus Creator/1 -> c19/1  "c19"

== system proc_control/Ros Command/Get_ROS_param/MPC Parameters/MPC Gains/Gains No DVL ==
  Bus Creator : BusCreator  Inputs=1
  MATLAB System5 : MATLABSystem  System=Vector2DoubleArray  arraySize=[1 MPC.nu]  constantName='No DVL MV'  SimulateUsing=Code generation
      mask Type: Vector2DoubleArray
      mask Display:
      | disp('Vector2DoubleArray');
      | port_label('input',1,'vector');
      | port_label('input',2,'length');
      | port_label('output',1,'array');
  MV : ros2lib/Get Parameter  ParameterName=proc_control.mpc.gains.noDvl.mv  ParameterType=double[]  ParameterMaxArrayLength=64  ParameterInitialValue=uint8([30,30,30,45,45,45,45,0])  SampleTime=-1  ModelName=proc_control  BlockId=ParamGet_proc_control_133
  noDvl : Outport
  wires:
  MV/2 -> MATLAB System5/2
  MV/1 -> MATLAB System5/1
  MATLAB System5/1 -> Bus Creator/1  "MV"
  Bus Creator/1 -> noDvl/1  "noDvl"

== matlab function proc_control/Subsystem ProcNav/SLAM Measurements/MATLAB Function ==
  data: u input; y output
function y = Normalize(u)

%Normailse le quaternions pour éviter la distortions crée par l'erreur de
% de l'intégration.
%q=quaternion(u(1), u(2), u(3), u(4));
d=norm(u);
n=u/d;
if isnan(n)
    y=[1;0;0;0];
else
    y = n;
end

== matlab function proc_control/Subsystem ProcNav/SLAM Measurements/MATLAB Function1 ==
  data: u input; y output
function y = Normalize(u)

%Normailse le quaternions pour éviter la distortions crée par l'erreur de
% de l'intégration.
%q=quaternion(u(1), u(2), u(3), u(4));
d=norm(u);
n=u/d;
if isnan(n)
    y=[1;0;0;0];
else
    y = n;
end

== matlab function proc_control/Subsystem ProcNav/AHRS//Detph Mesurments/MATLAB Function ==
  data: u input; y output
function y = Normalize(u)

%Normailse le quaternions pour éviter la distortions crée par l'erreur de
% de l'intégration.
%q=quaternion(u(1), u(2), u(3), u(4));
d=norm(u);
n=u/d;
if isnan(n)
    y=[1;0;0;0];
else
    y = n;
end

== matlab function proc_control/Subsystem ProcNav/DVL Measurements/MATLAB Function ==
  data: vBot input; v output; vWater input; thres input; error output; enable output
function [v, error, enable] = DVLManager(vBot,vWater,thres)

    if max(abs(vBot(1:3)))< thres
        %retouner les vitesse du bottom tracking (normal)
        v = vBot(1:3);
        enable = 1;
        error = ones(1,3) * vBot(4);
    elseif max(abs(vWater))< thres
        % retouner les vitesse du water profiling si bottom tracking fail
        v = vWater(1:3);
        enable = 0;
        error = ones(1,3) * vWater(4);
    else
        % Désactiver le dvl si mauvais data
        v = zeros(3,1);
        v(3)= 0;% patch(2);
        enable = 0;
        error = ones(1,3) * vBot(4);
    end
end

== matlab function proc_control/Subsystem Trajectory/SpaceNav/MATLAB Function ==
  data: matrix input; y output; p input
function y = fcn(matrix,p)
%matrix(10)=-matrix(10);
y = repmat(matrix,10,1);

== matlab function proc_control/Subsystem Trajectory/IDLE/MATLAB Function ==
  data: matrix input; y output; p input
function y = fcn(matrix,p)
matrix(10)=-matrix(10);
y = repmat(matrix,10,1);

== matlab function proc_control/Subsystem Controller/Controller List/If Action Subsystem1/MATLAB Function ==
  data: u input; A output; ysec input; Ts input; M input; x input; B output; C output; D output; U output; Y output; X output; DX output
function [A,B,C,D,U,Y,X,DX] = LtvTrimPlantQuat(u,ysec,Ts,M,x)

% Déterminer les dimentions
    nx = size(ysec,2);
    nu = size(u,2);
    p = size(u,1);

% Initialiser les matrices
    A = zeros(nx, nx, p);
    B = zeros(nx, nu, p);
    C = zeros(nx, nx, p);
    D = zeros(nx, nu, p);
    U = zeros(nu, 1, p);
    Y = zeros(13, 1, p);
    X = zeros(13, 1, p);
    DX = zeros(13, 1, p);
    
    
    xkk = x;
for i=1:p
    
    % Actualiser les états
        %xk=ysec(i,:).';
       
            xk=xkk;
      
        
        uk=u(i,:).';
        
    % Lineariser le model dynamique
        [Ac, Bc, C(:,:,i), D(:,:,i)]=AUV8QuatJacobianMatrix(xk,uk);


    % Generate discrete-time model
        A(:,:,i) = expm(Ac*Ts); % Fossen(2021) Eq B.10/B.9 page 662

        BT = Ac(8:13,8:13)\(A(8:13,8:13)-eye(6))*Bc(8:13,1:8); % Fossen(2021) Eq B.11 p 662
        B(:,:,i) = [zeros(7,8); BT];

    % Compute F(x(k+1),u)
       % xkk = ysec()
        % Intégration avec Euler Explicite
        for j=1:M 
          xkk = xkk + AUV8QuatSimFcn(xkk,uk)*(Ts/M);  
          % correct Quaternion
          d=norm(xkk(4:7));
          xkk(4:7) = xkk(4:7)./d;
        end

    % Nominal conditions for discrete-time plant
        U(:,:,i)  = uk.';
        Y(:,:,i)  = xk.';%(Cc*x + Dc*u).';
        X(:,:,i)  = xk.';
        DX(:,:,i) = (xkk-xk).' ;
       
end
disp(X)
end

== matlab function proc_control/Model System/Modele Thruster (Approximation)/MATLAB Function ==
  data: u input; y output
function y = wrapPWM(u)
 for i=1: size(u,1)
     if u(i)<1100 || u(i)>1900
         u(i)=1500;
     end
 end
y = u;

== matlab function proc_control/Model System/Quaternion Normalise ==
  data: u input; y output
function y = Normalize(u)
%Normailse le quaternions pour éviter la distortions crée par l'erreur de
% de l'intégration.
d=norm(u);
y = u/d;

== matlab function proc_control/Model System/Sensor Model/MATLAB Function ==
  data: epsilon input; y output; v input
function y = DvlLost(epsilon,v)
% This fonction simulate a ping failure if the pitch or roll angle is
% to important

e =abs(quat2eul(epsilon.','ZYX'));

if(e(2)>0.349066 || e(3)>0.349066) % If roll pitch exeed 20deg
    
    v = 32.7675*ones(3,1);
    
end

y = v;

== matlab function proc_control/Ros Command/Get_ROS_param/Physics Constants/MATLAB Function ==
  data: vec input; array output; length input
function array= fcn(vec, length)
array = zeros(8,6);
for i=1 : 8
    base_index = ((i-1)*6);
    array(i,:) = vec(base_index+1:base_index+6);
end
